simulink model "PID_without_security"  (R2021b)
settings: Solver=FixedStepAuto  StartTime=0.0  StopTime=8000  FixedStep=1
libraries: dspsigops x2, dspswit3 x2, slpidlib x1
settings Model: Creator=Karel  LastModifiedBy=HP
settings SolverCC: AlgebraicLoopSolver=TrustRegion
settings DataIOCC: ReturnWorkspaceOutputs=off
settings DebuggingCC: SFMachineParentedDataDiag=warning  ArithmeticOperatorsInVariantConditions=warning
settings SFSimCC: SimUseLocalCustomCode=off  CustomCodeUndefinedFunction=UseInterfaceOnly
settings RTWCC: RTWUseLocalCustomCode=off

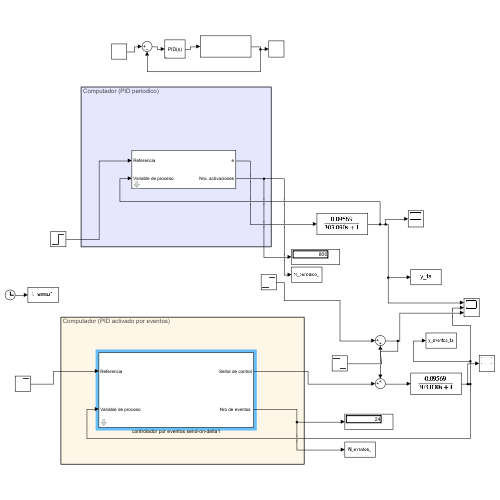
[thumbnail: Simulink's stored preview of the top-level diagram]
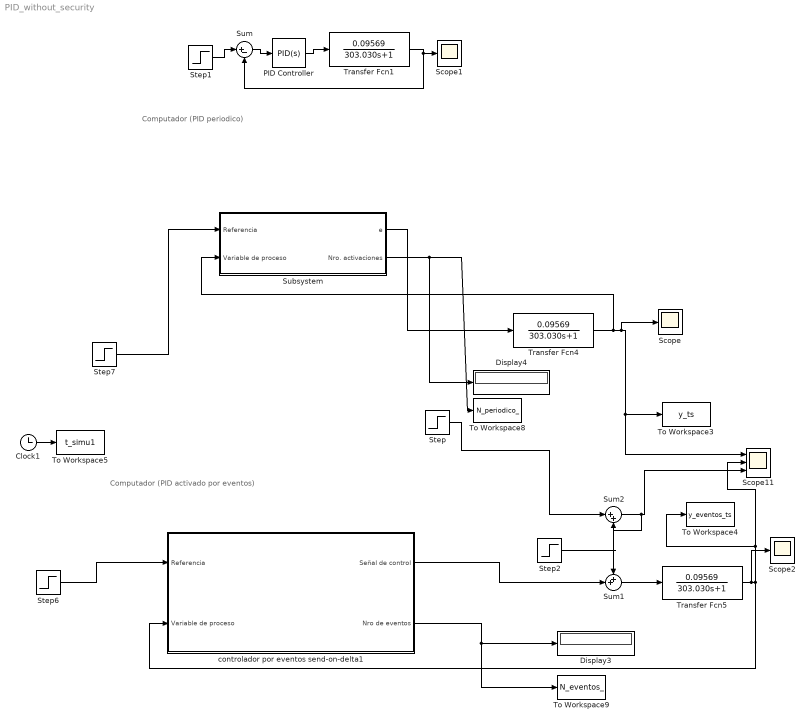
== system PID_without_security ==
  note: Computador (PID activado por eventos)
  note: Computador (PID periodico)
  Clock1 : Clock
  Display3 : Display
  Display4 : Display
  PID Controller : slpidlib/PID Controller  Controller=PID  Form=Parallel  TimeDomain=Continuous-time  UseExternalTs=off  SampleTime=-1  IntegratorMethod=Forward Euler  FilterMethod=Forward Euler  ControllerParametersSource=internal  P=100  I=5  D=0  UseFilter=on  N=100  TunerSelectOption=Transfer Function Based (PID Tuner App)  InitialConditionSource=internal  InitialConditionForIntegrator=0  InitialConditionForFilter=0  DifferentiatorICPrevScaledInput=0  ExternalReset=none  TrackingMode=off  Kt=1  LimitOutput=off  SatLimitsSource=internal  UpperSaturationLimit=inf  LowerSaturationLimit=-inf  LinearizeAsGain=on  AntiWindupMode=none  Kb=1  POutMin=[]  POutMax=[]  IOutMin=[]  IOutMax=[]  DOutMin=[]  DOutMax=[]  NOutMin=[]  NOutMax=[]  SumOutMin=[]  SumOutMax=[]  SaturationOutMin=[]  SaturationOutMax=[]  PParamMin=[]  PParamMax=[]  IParamMin=[]  IParamMax=[]  DParamMin=[]  DParamMax=[]  NParamMin=[]  NParamMax=[]  KbParamMin=[]  KbParamMax=[]  KtParamMin=[]  KtParamMax=[]  KbOutMin=[]  KbOutMax=[]  KtOutMin=[]  KtOutMax=[]  IntegratorOutMin=[]  IntegratorOutMax=[]  FilterOutMin=[]  FilterOutMax=[]  SumI1OutMin=[]  SumI1OutMax=[]  SumI2OutMin=[]  SumI2OutMax=[]  SumI3OutMin=[]  SumI3OutMax=[]  SumI4OutMin=[]  SumI4OutMax=[]  SumDOutMin=[]  SumDOutMax=[]  DifferentiatorOutMin=[]  DifferentiatorOutMax=[]  FilterDiffOutCoefMin=[]  FilterDiffOutCoefMax=[]  ReciprocalOutMin=[]  ReciprocalOutMax=[]  SumDenOutMin=[]  SumDenOutMax=[]  SumNumOutMin=[]  SumNumOutMax=[]  DivideOutMin=[]  DivideOutMax=[]  UdiffTsProdOutMin=[]  UdiffTsProdOutMax=[]  NTsProdOutMin=[]  NTsProdOutMax=[]  UintegralTsProdOutMin=[]  UintegralTsProdOutMax=[]  UngainTsProdOutMin=[]  UngainTsProdOutMax=[]  IntegratorContinuousStateAttributes=''  IntegratorStateMustResolveToSignalObject=off  IntegratorRTWStateStorageClass=Auto  FilterContinuousStateAttributes=''  FilterStateMustResolveToSignalObject=off  FilterRTWStateStorageClass=Auto  ParallelPVariant=InternalParameters  IdealPVariant=Disabled  IVariant=InternalParameters  DVariant=InternalParameters  IntegratorVariant=Continuous  SatVariant=Disabled  AWVariant=Passthrough  PCopyVariant=Disabled  TRVariant=Disabled  FdbkBlocksVariant=Forward  IdealPFdbkVariant=Disabled  SatFdbkVariant=Disabled  DerivativeFilterVariant=ContFilter  NVariant=InternalParameters  NCopyVariant=Disabled  FilterICVariant=InternalICsFilter  IntegratorICVariant=InternalICs  ExternalResetVariant=Disabled  TRSumVariant=Passthrough  SumFdbkVariant=Disabled  SumVariant=Sum_PID  TsampFilterVariant=InternalTs  TsampNgainVariant=Passthrough  TsampIntegralVariant=Passthrough  ExternalSaturationOutDataTypeStr=Inherit: Same as second input
  Scope : Scope
  Scope1 : Scope
  Scope11 : Scope  NumInputPorts=3
  Scope2 : Scope
  Step : Step  Time=3000  After=+10  SampleTime=0
  Step1 : Step  Time=0  SampleTime=0
  Step2 : Step  Time=3050  After=-10  SampleTime=0
  Step6 : Step  Time=0  SampleTime=0
  Step7 : Step  Time=0  SampleTime=0
  Subsystem : Subsystem  mask{Kp=33, Ki=0.181, Kd=0, N=100, Ts=10}
  Sum : Sum  Inputs=|+-
  Sum1 : Sum  Inputs=++|
  Sum2 : Sum  Inputs=|++
  To Workspace3 : ToWorkspace  VariableName=y_ts  SaveFormat=Structure With Time  SampleTime=-1
  To Workspace4 : ToWorkspace  VariableName=y_eventos_ts  SaveFormat=Structure With Time  SampleTime=-1
  To Workspace5 : ToWorkspace  VariableName=t_simu1  SampleTime=-1
      settings: Save2DSignal=2-D array (concatenate along first dimension)
  To Workspace8 : ToWorkspace  VariableName=N_periodico_  SampleTime=-1
      settings: Save2DSignal=2-D array (concatenate along first dimension)
  To Workspace9 : ToWorkspace  VariableName=N_eventos_  SampleTime=-1
      settings: Save2DSignal=2-D array (concatenate along first dimension)
  Transfer Fcn1 : TransferFcn  Numerator=[0.09569]  Denominator=[303.030 1]
  Transfer Fcn4 : TransferFcn  Numerator=[0.09569]  Denominator=[303.030 1]
  Transfer Fcn5 : TransferFcn  Numerator=[0.09569]  Denominator=[303.030 1]
  controlador por eventos send-on-delta1 : Subsystem  mask{Kp=33, Ki=0.181, Kd=0, N=100, elim=0.04, Ts=10, hmax=200}
      mask prompts: elim "Umbral de activacion"; hmax "Periodo max"
  wires:
  Step7/1 -> Subsystem/1(Referencia)
  Subsystem/2(Nro. activaciones) -> Display4/1, To Workspace8/1
  Subsystem/1(e) -> Transfer Fcn4/1
  Clock1/1 -> To Workspace5/1
  Transfer Fcn4/1 -> Scope11/1, To Workspace3/1, Scope/1, Subsystem/2(Variable de proceso)
  PID Controller/1 -> Transfer Fcn1/1
  Step1/1 -> Sum/1
  Sum/1 -> PID Controller/1
  Transfer Fcn1/1 -> Scope1/1, Sum/2
  Sum1/1 -> Transfer Fcn5/1
  Step/1 -> Sum2/1
  Step2/1 -> Sum2/2
  Sum2/1 -> Scope11/3, Sum1/1
  Transfer Fcn5/1 -> controlador por eventos send-on-delta1/2(Variable de proceso), Scope11/2, To Workspace4/1, Scope2/1
  controlador por eventos send-on-delta1/2("Nro de eventos ") -> To Workspace9/1, Display3/1
  Step6/1 -> controlador por eventos send-on-delta1/1(Referencia)
  controlador por eventos send-on-delta1/1(Señal de control) -> Sum1/2

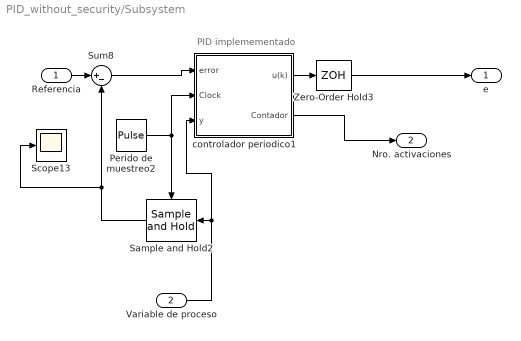
== system PID_without_security/Subsystem ==
  note: PID implemementado
  Referencia : Inport
  Variable de proceso : Inport  Port=2
  Perido de muestreo2 : DiscretePulseGenerator  PulseType=Time based  Period=Ts  PulseWidth=50
  Sample and Hold2 : dspsigops/Sample and Hold  trig=Rising edge  initCond=0  latchinput=off
  Scope13 : Scope
  Sum8 : Sum  Inputs=|+-
  Zero-Order Hold3 : ZeroOrderHold  SampleTime=-1
  controlador periodico1 : Subsystem
  e : Outport  VectorParamsAs1DForOutWhenUnconnected=off
  Nro. activaciones : Outport  Port=2  VectorParamsAs1DForOutWhenUnconnected=off
  wires:
  Sum8/1 -> controlador periodico1/1(error)
  Sample and Hold2/1 -> Sum8/2, Scope13/1
  Perido de muestreo2/1 -> controlador periodico1/2(Clock), Sample and Hold2/Trigger
  controlador periodico1/1(u(k)) -> Zero-Order Hold3/1
  controlador periodico1/2(Contador) -> Nro. activaciones/1
  Variable de proceso/1 -> controlador periodico1/3(y), Sample and Hold2/1
  Referencia/1 -> Sum8/1
  Zero-Order Hold3/1 -> e/1

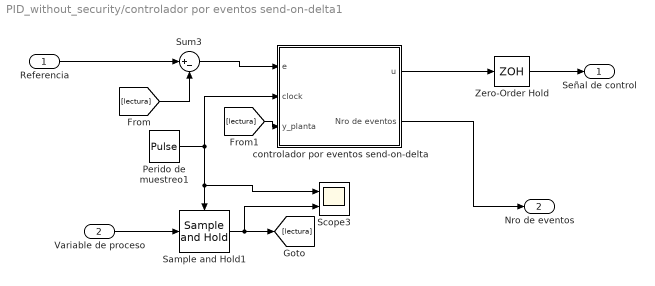
== system PID_without_security/controlador por eventos send-on-delta1 ==
  Referencia : Inport
  Variable de proceso : Inport  Port=2
  Perido de muestreo1 : DiscretePulseGenerator  PulseType=Time based  Period=Ts  PulseWidth=50
  Sample and Hold1 : dspsigops/Sample and Hold  trig=Rising edge  initCond=0  latchinput=off
  Scope3 : Scope  NumInputPorts=2
  Sum3 : Sum  Inputs=|+-
  Zero-Order Hold : ZeroOrderHold  SampleTime=-1
  controlador por eventos send-on-delta : Subsystem
  Señal de control : Outport
  "Nro de eventos " : Outport  Port=2
  wires:
  Perido de muestreo1/1 -> controlador por eventos send-on-delta/2(clock), Scope3/1, Sample and Hold1/Trigger
  Sum3/1 -> controlador por eventos send-on-delta/1(e)
  Sample and Hold1/1 -> Scope3/2, [lectura]
  [lectura] -> controlador por eventos send-on-delta/3(y_planta)
  Zero-Order Hold/1 -> Señal de control/1
  [lectura] -> Sum3/2
  controlador por eventos send-on-delta/1(u) -> Zero-Order Hold/1
  controlador por eventos send-on-delta/2("Nro de eventos ") -> "Nro de eventos "/1
  Variable de proceso/1 -> Sample and Hold1/1
  Referencia/1 -> Sum3/1

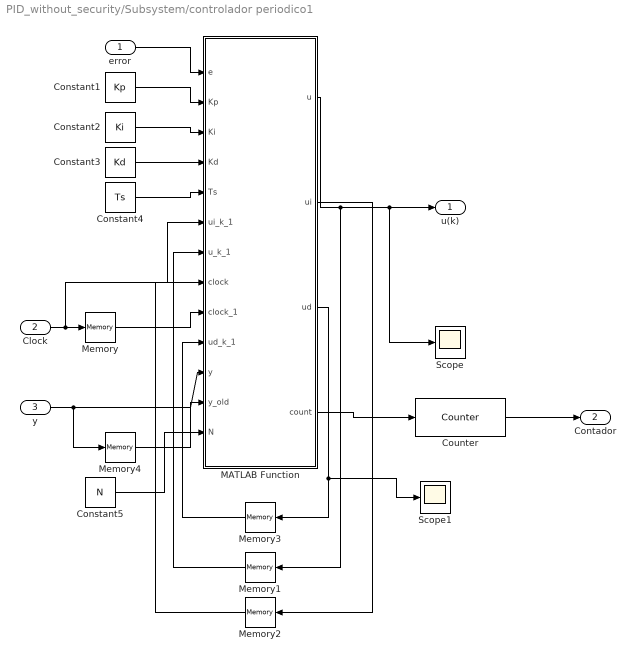
== system PID_without_security/Subsystem/controlador periodico1 ==
  error : Inport
  Clock : Inport  Port=2
  y : Inport  Port=3
  Constant1 : Constant  Value=Kp
  Constant2 : Constant  Value=Ki
  Constant3 : Constant  Value=Kd
  Constant4 : Constant  Value=Ts
  Constant5 : Constant  Value=N
  Counter : dspswit3/Counter  Direction=Up  CountEvent=Rising edge  CounterSize=User defined  MaxCount=20000  InitialCount=0  Output=Count  HitValue=32  ResetInput=off  SamplesPerFrame=1  Ts=1  CntDtype=double  HitDtype=Logical
  MATLAB Function : MATLAB Function  TreatAsAtomicUnit=on
  Memory{,1..4} (5 alike) : Memory
  Scope : Scope
  Scope1 : Scope
  u(k) : Outport  VectorParamsAs1DForOutWhenUnconnected=off
  Contador : Outport  Port=2  VectorParamsAs1DForOutWhenUnconnected=off
  wires:
  Counter/1 -> Contador/1
  MATLAB Function/4(count) -> Counter/1
  Constant4/1 -> MATLAB Function/5(Ts)
  Memory/1 -> MATLAB Function/9(clock_1)
  Clock/1 -> MATLAB Function/8(clock), Memory/1
  MATLAB Function/1(u) -> u(k)/1, Scope/1, Memory1/1
  Memory1/1 -> MATLAB Function/7(u_k_1)
  error/1 -> MATLAB Function/1(e)
  Constant1/1 -> MATLAB Function/2(Kp)
  Constant2/1 -> MATLAB Function/3(Ki)
  Memory2/1 -> MATLAB Function/6(ui_k_1)
  MATLAB Function/2(ui) -> Memory2/1
  MATLAB Function/3(ud) -> Scope1/1, Memory3/1
  Memory3/1 -> MATLAB Function/10(ud_k_1)
  y/1 -> Memory4/1, MATLAB Function/11(y)
  Memory4/1 -> MATLAB Function/12(y_old)
  Constant3/1 -> MATLAB Function/4(Kd)
  Constant5/1 -> MATLAB Function/13(N)

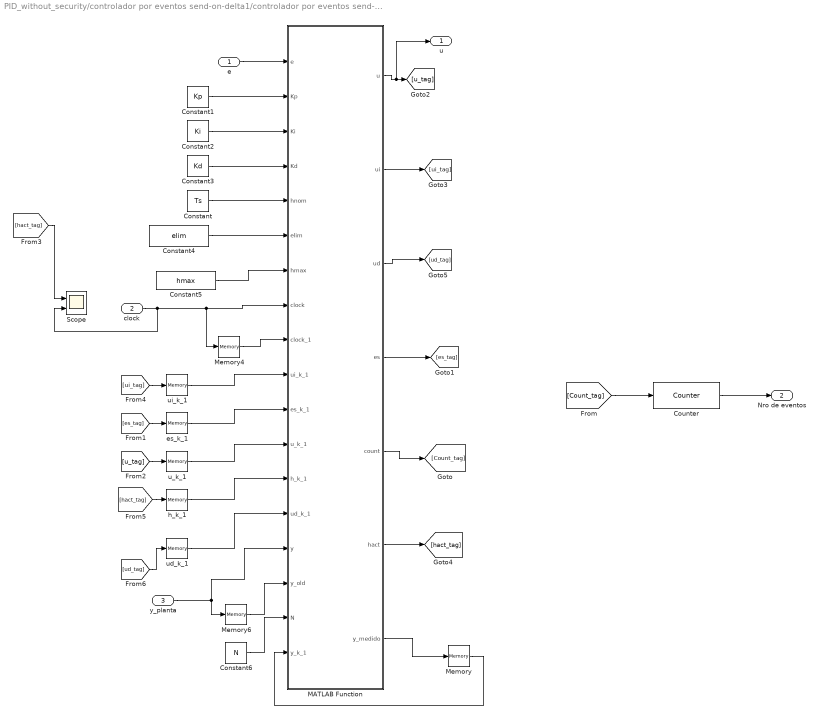
== system PID_without_security/controlador por eventos send-on-delta1/controlador por eventos send-on-delta ==
  e : Inport
  clock : Inport  Port=2
  y_planta : Inport  Port=3
  Constant : Constant  Value=Ts
  Constant1 : Constant  Value=Kp
  Constant2 : Constant  Value=Ki
  Constant3 : Constant  Value=Kd
  Constant4 : Constant  Value=elim
  Constant5 : Constant  Value=hmax
  Constant6 : Constant  Value=N
  Counter : dspswit3/Counter  Direction=Up  CountEvent=Rising edge  CounterSize=User defined  MaxCount=20000  InitialCount=0  Output=Count  HitValue=32  ResetInput=off  SamplesPerFrame=1  Ts=1  CntDtype=double  HitDtype=Logical
  MATLAB Function : MATLAB Function  TreatAsAtomicUnit=on
  Memory : Memory
  Memory4 : Memory
  Memory6 : Memory
  Scope : Scope  NumInputPorts=2
  es_k_1 : Memory
  h_k_1 : Memory
  u_k_1 : Memory
  ud_k_1 : Memory
  ui_k_1 : Memory
  u : Outport  VectorParamsAs1DForOutWhenUnconnected=off
  "Nro de eventos " : Outport  Port=2  VectorParamsAs1DForOutWhenUnconnected=off
  wires:
  ui_k_1/1 -> MATLAB Function/10(ui_k_1)
  Constant2/1 -> MATLAB Function/3(Ki)
  Constant1/1 -> MATLAB Function/2(Kp)
  e/1 -> MATLAB Function/1(e)
  Constant/1 -> MATLAB Function/5(hnom)
  Constant4/1 -> MATLAB Function/6(elim)
  u_k_1/1 -> MATLAB Function/12(u_k_1)
  es_k_1/1 -> MATLAB Function/11(es_k_1)
  h_k_1/1 -> MATLAB Function/13(h_k_1)
  Counter/1 -> "Nro de eventos "/1
  Memory4/1 -> MATLAB Function/9(clock_1)
  y_planta/1 -> Memory6/1, MATLAB Function/15(y)
  Memory6/1 -> MATLAB Function/16(y_old)
  MATLAB Function/5(count) -> [Count_tag]
  [Count_tag] -> Counter/1
  MATLAB Function/4(es) -> [es_tag]
  [es_tag] -> es_k_1/1
  [u_tag] -> u_k_1/1
  MATLAB Function/1(u) -> u/1, [u_tag]
  MATLAB Function/2(ui) -> [ui_tag]
  [ui_tag] -> ui_k_1/1
  MATLAB Function/6(hact) -> [hact_tag]
  [hact_tag] -> h_k_1/1
  MATLAB Function/3(ud) -> [ud_tag]
  [ud_tag] -> ud_k_1/1
  ud_k_1/1 -> MATLAB Function/14(ud_k_1)
  Constant3/1 -> MATLAB Function/4(Kd)
  Constant5/1 -> MATLAB Function/7(hmax)
  Constant6/1 -> MATLAB Function/17(N)
  Memory/1 -> MATLAB Function/18(y_k_1)
  MATLAB Function/7(y_medido) -> Memory/1
  [hact_tag] -> Scope/1
  clock/1 -> Scope/2, Memory4/1, MATLAB Function/8(clock)

== matlab function PID_without_security/Subsystem/controlador periodico1/MATLAB Function ==
  data: e input; u output; Kp input; Ki input; Kd input; Ts input; ui_k_1 input; ui output; ud output; u_k_1 input; clock input; clock_1 input; count output; ud_k_1 input; y input; y_old input; N input
function [u,ui,ud,count]  = fcn(e,Kp,Ki,Kd,Ts,ui_k_1,u_k_1,clock,clock_1,ud_k_1,y,y_old,N)
if(clock==1 && clock_1==0)
    %Ejecución del algoritmo de PID
    up=Kp*(e);              %Acción proporcional
    ud=(Kd/(Kd+N*Kp*Ts))*(ud_k_1-Kp*N*(y-y_old));
    u=up + ui_k_1 + ud;          %Generación de señal de control
    
    %Calculo de acción integral en tk+1
    ui=ui_k_1 + (Ki*Ts)*(e);
    
    %Contador de ejecuciones del algoritmo PID
    count=1;
else
    u=u_k_1;                
    ui=ui_k_1;
    ud=ud_k_1;
    count=0;
end

== matlab function PID_without_security/controlador por eventos send-on-delta1/controlador por eventos send-on-delta/MATLAB Function ==
  data: e input; u output; Kp input; Ki input; Kd input; hnom input; elim input; hmax input; clock input; clock_1 input; ui_k_1 input; ui output; ud output; es_k_1 input; es output; u_k_1 input; count output; h_k_1 input; ud_k_1 input; y input; hact output; y_old input; N input; y_k_1 input; y_medido output
function [u,ui,ud,es,count,hact,y_medido]  = fcn(e,Kp,Ki,Kd,hnom,elim,hmax,clock,clock_1,ui_k_1,es_k_1,u_k_1,h_k_1,ud_k_1,y,y_old,N,y_k_1)
if(clock==1 && clock_1==0)
    hact=h_k_1 + hnom;      %Cálculo del periodo de muestreo actual
    
    if(abs(e-es_k_1)>elim)    %Condición de umbrales de activación
       es=e;        %Actualización del valor de error de es                          
       %Ejecución del algoritmo de PID
       up=Kp*(e);   %Accion proporcional
       ud=(Kd/(Kd+N*Kp*hact))*(ud_k_1 - Kp*N*(y-y_old));
       if(hact >=hmax)
           hexp = hact*exp(hnom-hact);
           E = (hexp - hnom)*elim + hnom*e;
       else
           E = hact*e;
       end    
       ui=ui_k_1 + Ki*E;
       u=up + ui + ud;
       hact=0;
       
       %Contador de ejecuciones del algoritmo PID
       count=1; 
       y_medido = y;
       
    else
       %Si no existe evento, las variables no cambian
       u=u_k_1; 
       ui=ui_k_1;
       ud=ud_k_1;
       es=es_k_1;
       count=0;
       y_medido = y_k_1;
    end  
    
else
   u=u_k_1; 
   ui=ui_k_1;
   ud=ud_k_1;
   es=es_k_1;
   count=0;
   hact=h_k_1;
   y_medido = y_k_1;
end
